simulink model "pid"  (Simulink 7.5)
settings: Solver=ode45  StartTime=0.0  StopTime=100  RelTol=1e-3
undefined symbols (not defined in the file): b, c, Kr, Td, Tdf, Ti, Tt, yref
settings Model: Creator=sieklo  LastModifiedBy=Konrad

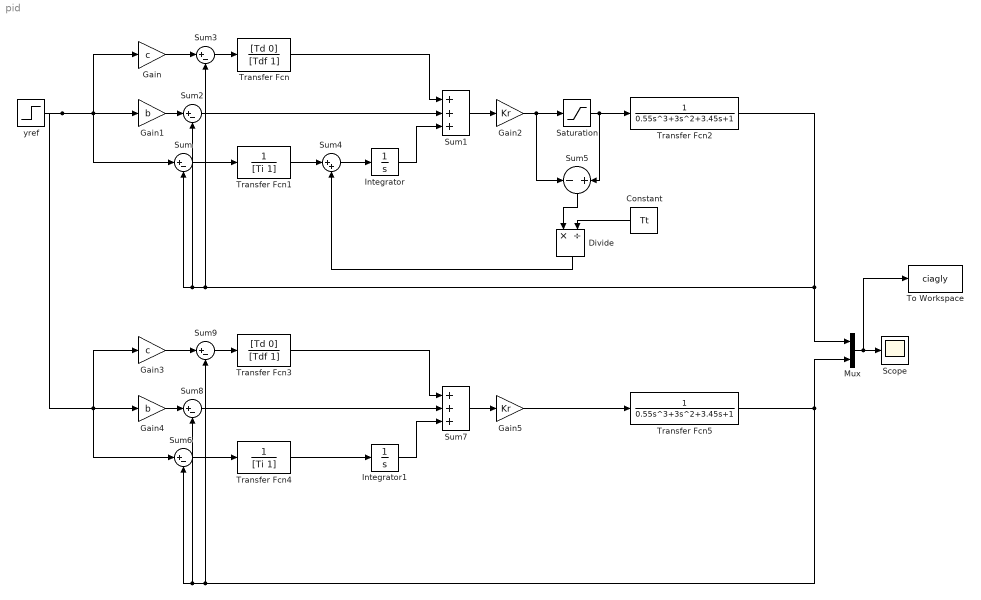
== system pid ==
  Constant : Constant  Value=Tt
  Divide : Product  Inputs=*/
  Gain : Gain  Gain=c
  Gain1 : Gain  Gain=b
  Gain2 : Gain  Gain=Kr
  Gain3 : Gain  Gain=c
  Gain4 : Gain  Gain=b
  Gain5 : Gain  Gain=Kr
  Integrator : Integrator
  Integrator1 : Integrator
  Mux : Mux  Inputs=2
  Saturation : Saturate
  Scope : Scope
  Sum{,2..3,6,8..9} (6 alike) : Sum  Inputs=|+-
  Sum1 : Sum  Inputs=+++
  Sum4 : Sum  Inputs=|++
  Sum5 : Sum  Inputs=-+
  Sum7 : Sum  Inputs=+++
  To Workspace : ToWorkspace  VariableName=ciagly  SampleTime=-1  SaveFormat=Structure
  Transfer Fcn : TransferFcn  Numerator=[Td 0]  Denominator=[Tdf 1]
  Transfer Fcn1 : TransferFcn  Denominator=[Ti 1]
  Transfer Fcn2 : TransferFcn  Denominator=[0.55 3 3.45 1]
  Transfer Fcn3 : TransferFcn  Numerator=[Td 0]  Denominator=[Tdf 1]
  Transfer Fcn4 : TransferFcn  Denominator=[Ti 1]
  Transfer Fcn5 : TransferFcn  Denominator=[0.55 3 3.45 1]
  yref : Step  After=yref  SampleTime=0
  wires:
  Sum/1 -> Transfer Fcn1/1
  Transfer Fcn/1 -> Sum1/1
  Sum3/1 -> Transfer Fcn/1
  Gain/1 -> Sum3/1
  yref/1 -> Gain1/1, Gain/1, Sum/1, Gain4/1, Gain3/1, Sum6/1
  Gain1/1 -> Sum2/1
  Sum2/1 -> Sum1/2
  Sum4/1 -> Integrator/1
  Transfer Fcn1/1 -> Sum4/1
  Integrator/1 -> Sum1/3
  Saturation/1 -> Sum5/2, Transfer Fcn2/1
  Gain2/1 -> Saturation/1, Sum5/1
  Sum1/1 -> Gain2/1
  Transfer Fcn2/1 -> Sum/2, Sum2/2, Sum3/2, Mux/1
  Divide/1 -> Sum4/2
  Sum5/1 -> Divide/1
  Constant/1 -> Divide/2
  Sum6/1 -> Transfer Fcn4/1
  Transfer Fcn3/1 -> Sum7/1
  Sum9/1 -> Transfer Fcn3/1
  Gain3/1 -> Sum9/1
  Gain4/1 -> Sum8/1
  Sum8/1 -> Sum7/2
  Transfer Fcn4/1 -> Integrator1/1
  Integrator1/1 -> Sum7/3
  Gain5/1 -> Transfer Fcn5/1
  Sum7/1 -> Gain5/1
  Transfer Fcn5/1 -> Sum6/2, Sum8/2, Sum9/2, Mux/2
  Mux/1 -> Scope/1, To Workspace/1
